simulink model "casper_sim_phase0_legacy"  (R2025b)
settings: Solver=FixedStepDiscrete  StartTime=0  StopTime=549  FixedStep=1e-4  RelTol=1e-3
libraries: casper_sim_lib x1
settings Model: Creator=Ashwin  LastModifiedBy=Ashwin

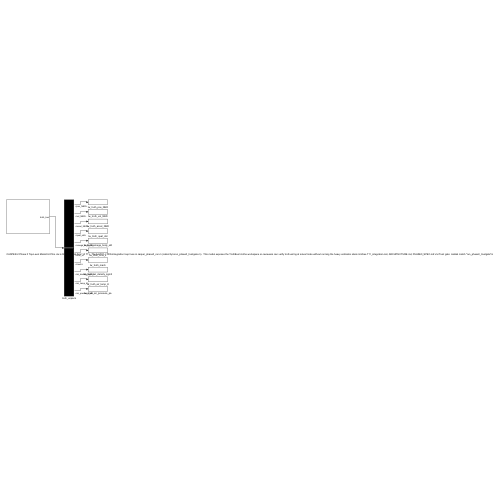
[thumbnail: Simulink's stored preview of the top-level diagram]
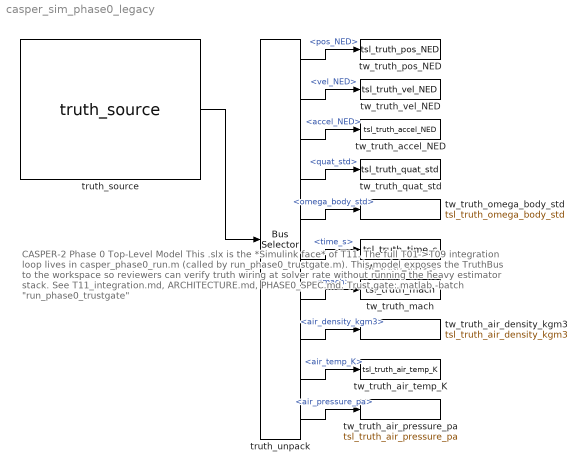
== system casper_sim_phase0_legacy ==
  note: CASPER-2 Phase 0 Top-Level Model\n\nThis .slx is the *Simulink face* of T11. The full T01->T09\nintegration loop lives in casper_phase0_run.m (called by\nrun_phase0_trustgate.m). This model exposes the TruthBus to\nthe workspace so reviewers can verify truth wiring at solver\nrate without running the heavy estimator stack.\n\nSee T11_integration.md, ARCHITECTURE.md, PHASE0_SPEC.md.\n\nTrust gate: matlab -batch "run_phase0_trustgate"\n
  truth_source : casper_sim_lib/truth_source  SystemSampleTime=-1  VariantActivationTime=update diagram  EmptyChoice=off  PassThrough=off  PassThroughVariantControl=(default)  EmptyChoiceVariantControl=(default)  AllowFlexibleInterface=on  Latency=0  AutoFrameSizeCalculation=off
  truth_unpack : BusSelector  OutputSignals=pos_NED,vel_NED,accel_NED,quat_std,omega_body_std,time_s,mach,air_density_kgm3,air_temp_K,air_pressure_pa
  tw_truth_accel_NED : ToWorkspace  VariableName=tsl_truth_accel_NED  SaveFormat=Timeseries  SampleTime=-1
  tw_truth_air_density_kgm3 : ToWorkspace  VariableName=tsl_truth_air_density_kgm3  SaveFormat=Timeseries  SampleTime=-1
  tw_truth_air_pressure_pa : ToWorkspace  VariableName=tsl_truth_air_pressure_pa  SaveFormat=Timeseries  SampleTime=-1
  tw_truth_air_temp_K : ToWorkspace  VariableName=tsl_truth_air_temp_K  SaveFormat=Timeseries  SampleTime=-1
  tw_truth_mach : ToWorkspace  VariableName=tsl_truth_mach  SaveFormat=Timeseries  SampleTime=-1
  tw_truth_omega_body_std : ToWorkspace  VariableName=tsl_truth_omega_body_std  SaveFormat=Timeseries  SampleTime=-1
  tw_truth_pos_NED : ToWorkspace  VariableName=tsl_truth_pos_NED  SaveFormat=Timeseries  SampleTime=-1
  tw_truth_quat_std : ToWorkspace  VariableName=tsl_truth_quat_std  SaveFormat=Timeseries  SampleTime=-1
  tw_truth_time_s : ToWorkspace  VariableName=tsl_truth_time_s  SaveFormat=Timeseries  SampleTime=-1
  tw_truth_vel_NED : ToWorkspace  VariableName=tsl_truth_vel_NED  SaveFormat=Timeseries  SampleTime=-1
  wires:
  truth_source/1 -> truth_unpack/1
  truth_unpack/1 -> tw_truth_pos_NED/1  "<pos_NED>"
  truth_unpack/2 -> tw_truth_vel_NED/1  "<vel_NED>"
  truth_unpack/3 -> tw_truth_accel_NED/1  "<accel_NED>"
  truth_unpack/4 -> tw_truth_quat_std/1  "<quat_std>"
  truth_unpack/5 -> tw_truth_omega_body_std/1  "<omega_body_std>"
  truth_unpack/6 -> tw_truth_time_s/1  "<time_s>"
  truth_unpack/7 -> tw_truth_mach/1  "<mach>"
  truth_unpack/8 -> tw_truth_air_density_kgm3/1  "<air_density_kgm3>"
  truth_unpack/9 -> tw_truth_air_temp_K/1  "<air_temp_K>"
  truth_unpack/10 -> tw_truth_air_pressure_pa/1  "<air_pressure_pa>"
